simulink model "aeroelastic_control_updated_2023a"  (R2023a)
settings: Solver=FixedStepAuto  StartTime=0.0  StopTime=100  FixedStep=0.001  RelTol=1e-3
InitFcn:
  | A_ae = zeros(12);
  | B_ae = zeros(12,1);
  | C_ae = zeros(1,12);
model workspace (MAT data in the model file):
  C_L = 5
  delta = 5
  k_a = 1
  k_alpha = 4
  k_h = 1
  m = 15.91
  x_cg = 0.35
  x_ea = 0.45
libraries: simulink x1
settings Model: Creator=adrianbuda  LastModifiedBy=divij
settings DataIOCC: SaveFormat=Structure
settings OptimizationCC: DefaultParameterBehavior=Inlined  UseDivisionForNetSlopeComputation=on  GainParamInheritBuiltInType=on  UseFloatMulNetSlope=on  InlineInvariantSignals=on  ZeroExternalMemoryAtStartup=off  ZeroInternalMemoryAtStartup=off  EfficientFloat2IntCast=on  LifeSpan=1  OptimizeDataStoreBuffers=off  BusAssignmentInplaceUpdate=off
settings DebuggingCC: SFUnexpectedBacktrackingDiag=warning  SFNoUnconditionalDefaultTransitionDiag=warning
settings HardwareCC: ProdLongLongMode=on
settings SFSimCC: MATLABDynamicMemAlloc=off
settings RTWCC: PackageGeneratedCodeAndArtifacts=on  GenerateReport=on  Toolchain=Catkin  BuildConfiguration=Debug  LaunchReport=on  TargetLang=C++
settings CodeAppCC: ForceParamTrailComments=on  EnableCustomComments=on
settings GRTTargetCC: TargetLangStandard=C++11 (ISO)  CombineSignalStateStructs=on  MatFileLogging=off  CodeInterfacePackaging=C++ class  SupportVariableSizeSignals=on  MultiInstanceErrorCode=Warning

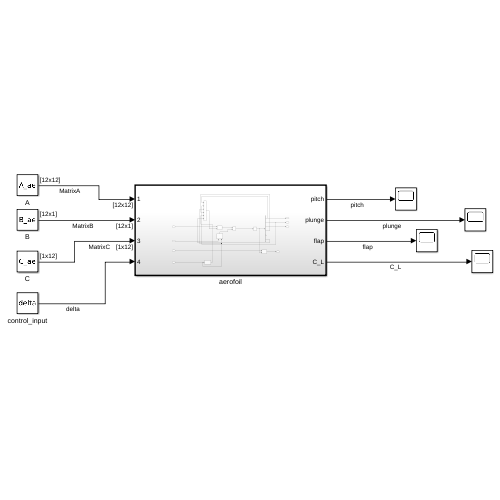
[thumbnail: Simulink's stored preview of the top-level diagram]
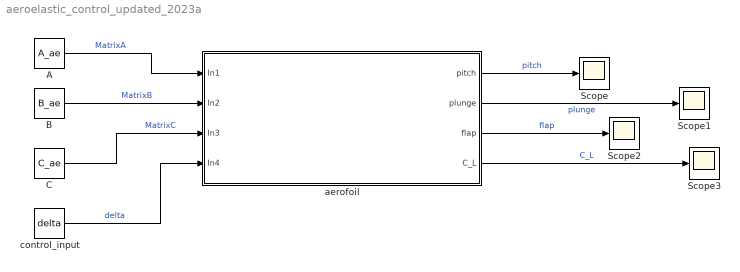
== system aeroelastic_control_updated_2023a ==
  A : Constant  Value=A_ae  VectorParams1D=off
  B : Constant  Value=B_ae  VectorParams1D=off
  C : Constant  Value=C_ae  VectorParams1D=off
  Scope{,1..3} (4 alike) : Scope
  aerofoil : Subsystem  TreatAsAtomicUnit=on
  control_input : Constant  Value=delta  VectorParams1D=off
  wires:
  A/1 -> aerofoil/1(In1)  "MatrixA"
  B/1 -> aerofoil/2(In2)  "MatrixB"
  C/1 -> aerofoil/3(In3)  "MatrixC"
  control_input/1 -> aerofoil/4(In4)  "delta"
  aerofoil/1(pitch) -> Scope/1  "pitch"
  aerofoil/2(plunge) -> Scope1/1  "plunge"
  aerofoil/3(flap) -> Scope2/1  "flap"
  aerofoil/4(C_L) -> Scope3/1  "C_L"

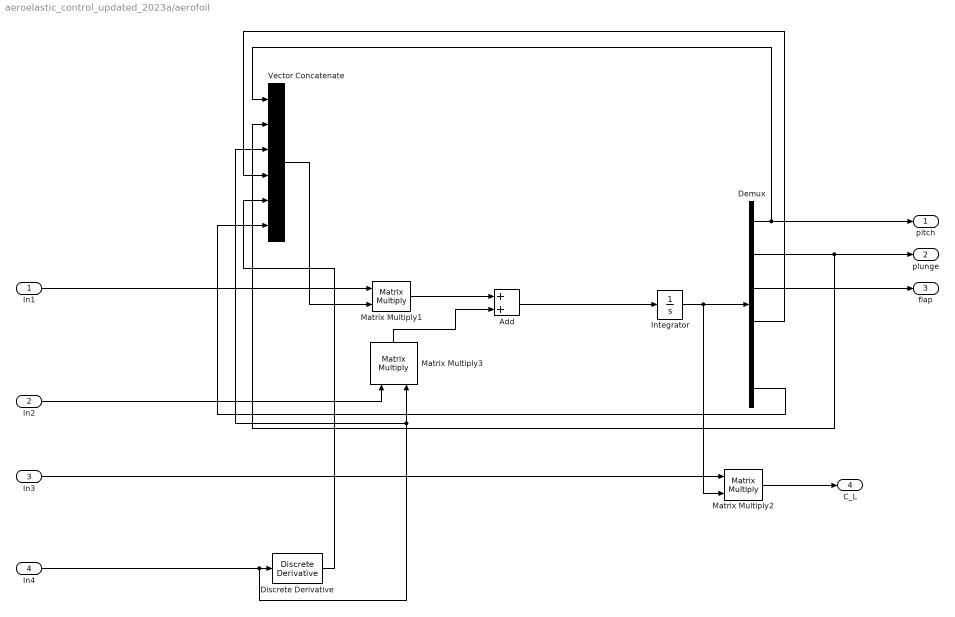
== system aeroelastic_control_updated_2023a/aerofoil ==
  In1 : Inport
  In2 : Inport  Port=2
  In3 : Inport  Port=3
  In4 : Inport  Port=4
  Add : Sum
  Demux : Demux  Outputs=[1,1,1,2,1,6]
  Discrete Derivative : simulink/Discrete/Discrete Derivative  gainval=1.0  ICPrevScaledInput=0.0  OutMin=[]  OutMax=[]  OutDataType=fixdt(1, 16)  OutScaling=2^-10  DoSatur=off
  Integrator : Integrator
  Matrix Multiply1 : Product  Multiplication=Matrix(*)
  Matrix Multiply2 : Product  Multiplication=Matrix(*)
  Matrix Multiply3 : Product  Multiplication=Matrix(*)
  Vector Concatenate : Concatenate  NumInputs=6
  pitch : Outport
  plunge : Outport  Port=2
  flap : Outport  Port=3
  C_L : Outport  Port=4
  wires:
  In4/1 -> Vector Concatenate/3, Matrix Multiply3/2, Discrete Derivative/1
  In1/1 -> Matrix Multiply1/1
  Demux/1 -> Vector Concatenate/1, pitch/1
  Integrator/1 -> Matrix Multiply2/2, Demux/1
  Demux/2 -> Vector Concatenate/2, plunge/1
  In3/1 -> Matrix Multiply2/1
  Demux/3 -> flap/1
  Discrete Derivative/1 -> Vector Concatenate/5
  In2/1 -> Matrix Multiply3/1
  Matrix Multiply2/1 -> C_L/1
  Add/1 -> Integrator/1
  Demux/4 -> Vector Concatenate/4
  Demux/6 -> Vector Concatenate/6
  Vector Concatenate/1 -> Matrix Multiply1/2
  Matrix Multiply1/1 -> Add/1
  Matrix Multiply3/1 -> Add/2
